simulink model "Controlled_Three_phase_full_wave_bridge_rectifier_PI"  (R2023b)
settings: Solver=VariableStepAuto  StartTime=0.0  StopTime=0.2  RelTol=1e-3
libraries: spsThyristorLib x6, spsSeriesRLCBranchLib x4, spsVoltageMeasurementLib x4, spsACVoltageSourceLib x3, spsCurrentMeasurementLib x1, sps_lib x1
settings Model: Creator=louis  LastModifiedBy=louis

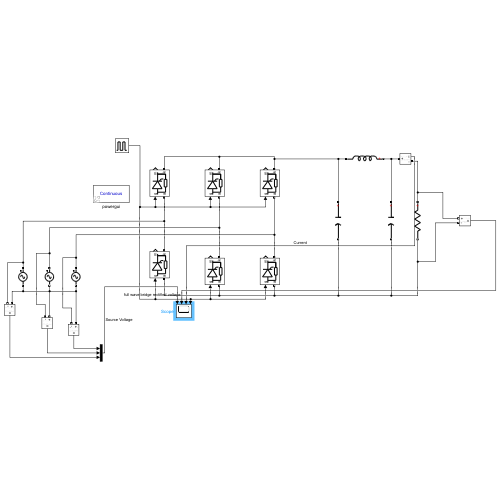
[thumbnail: Simulink's stored preview of the top-level diagram]
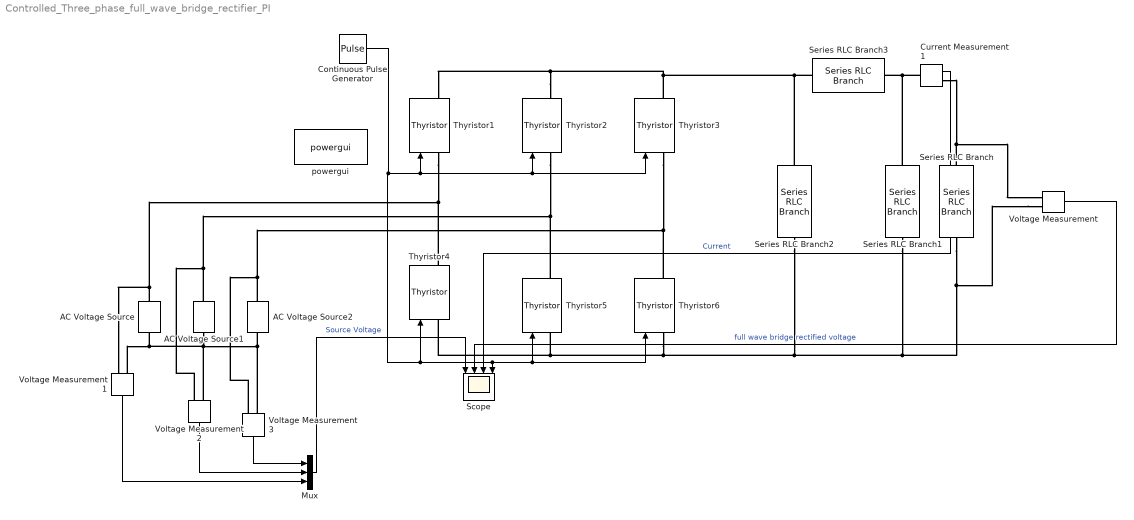
== system Controlled_Three_phase_full_wave_bridge_rectifier_PI ==
  AC Voltage Source : spsACVoltageSourceLib/AC Voltage Source  Amplitude=240  Phase=0  Frequency=50  SampleTime=0  Measurements=None  BusType=swing  Pref=10e3  Qref=0  Qmin=-inf  Qmax=+inf
  AC Voltage Source1 : spsACVoltageSourceLib/AC Voltage Source  Amplitude=240  Phase=120  Frequency=50  SampleTime=0  Measurements=None  BusType=swing  Pref=10e3  Qref=0  Qmin=-inf  Qmax=+inf
  AC Voltage Source2 : spsACVoltageSourceLib/AC Voltage Source  Amplitude=240  Phase=240  Frequency=50  SampleTime=0  Measurements=None  BusType=swing  Pref=10e3  Qref=0  Qmin=-inf  Qmax=+inf
  Continuous Pulse Generator : DiscretePulseGenerator  PulseType=Time based  Period=0.0033  PulseWidth=50  PhaseDelay=0.002
  Current Measurement1 : spsCurrentMeasurementLib/Current Measurement  PhasorSimulation=off  OutputType=Complex  PSBequivalent=0
  Mux : Mux  Inputs=3
  Scope : Scope  NumInputPorts=4
  Series RLC Branch : spsSeriesRLCBranchLib/Series RLC Branch  LConnTagsString=__new0  RConnTagsString=__new0  BranchType=R  Resistance=0.8  Inductance=0.001  SetiL0=off  InitialCurrent=0  Capacitance=1e-6  Setx0=off  InitialVoltage=0  Measurements=None
  Series RLC Branch1 : spsSeriesRLCBranchLib/Series RLC Branch  LConnTagsString=__new0  RConnTagsString=__new0  BranchType=C  Resistance=0.8  Inductance=0.001  SetiL0=off  InitialCurrent=0  Capacitance=0.000001  Setx0=off  InitialVoltage=0  Measurements=None
  Series RLC Branch2 : spsSeriesRLCBranchLib/Series RLC Branch  LConnTagsString=__new0  RConnTagsString=__new0  BranchType=C  Resistance=0.8  Inductance=0.001  SetiL0=off  InitialCurrent=0  Capacitance=0.000001  Setx0=off  InitialVoltage=0  Measurements=None
  Series RLC Branch3 : spsSeriesRLCBranchLib/Series RLC Branch  LConnTagsString=__new0  RConnTagsString=__new0  BranchType=L  Resistance=0.8  Inductance=0.003  SetiL0=off  InitialCurrent=0  Capacitance=0.1  Setx0=off  InitialVoltage=0  Measurements=None
  Thyristor{1..6} (6 alike) : spsThyristorLib/Thyristor  Ron=0.001  Lon=0  Vf=0.8  IC=0  Rs=500  Cs=250e-9  Measurements=on
  Voltage Measurement{,1..3} (4 alike) : spsVoltageMeasurementLib/Voltage Measurement  PhasorSimulation=off  OutputType=Complex  PSBequivalent=0
  powergui : sps_lib/powergui  Priority=1  SimulationMode=Continuous  SampleTime=50e-6  frequency=60  Iterations=50  frequencyindice=0  Pbase=100e6  ErrMax=1e-4  UnitsV=kV  UnitsW=MW  buscounter=0  FunctionMessages=off  echomessages=off  EnableUseOfTLC=off  CurrentSourceSwitches=off  DisableSnubberDevices=off  DisableRonSwitches=off  DisableVfSwitches=off  DisplayEquations=off  AutomaticDiscreteSolvers=off  SolverType=Tustin/Backward Euler (TBE)  Interpol=off  ExternalGateDelay=off  methode=off  Ts=100  x0status=blocks  SPID=on  SwTol=0  HookPort=off  NonlinearTolerance=1e-4  nMaxIteration=100  ContinueOnMaxIteration=off  RestoreLinks=warning  ResistiveCurrentMeasurement=off  Frange=[0:2:500]  Ylog=off  Xlog=on  ShowGrid=off  save=off  variable=ZData  structure=0  ZoomFFT=off  StartTime=0.0  cycles=1  DisplayStyle=1  fundamental=60  FreqAxis=off  MaxFrequency=1000  frequencyindicesteady=1  RmsSteady=1  display=off
  wires:
  Voltage Measurement/1 -> Scope/2  "full wave bridge rectified voltage"
  Voltage Measurement3/1 -> Mux/1
  Voltage Measurement2/1 -> Mux/2
  Voltage Measurement1/1 -> Mux/3
  Mux/1 -> Scope/1  "Source Voltage"
  Continuous Pulse Generator/1 -> Thyristor3/1, Thyristor2/1, Thyristor1/1, Thyristor4/1, Thyristor6/1, Thyristor5/1, Scope/4
  Current Measurement1/1 -> Scope/3  "Current"
  connections:
  Series RLC Branch1/LConn1 -- Series RLC Branch3/LConn1 -- Current Measurement1/LConn1
  Voltage Measurement1/LConn2 -- AC Voltage Source/RConn1 -- Thyristor4/RConn1 -- Thyristor1/LConn1
  Voltage Measurement2/LConn2 -- AC Voltage Source1/RConn1 -- Thyristor5/RConn1 -- Thyristor2/LConn1
  Voltage Measurement/LConn2 -- Series RLC Branch1/RConn1 -- Series RLC Branch2/RConn1 -- Thyristor6/LConn1 -- Thyristor4/LConn1 -- Thyristor5/LConn1 -- Series RLC Branch/RConn1
  Thyristor2/RConn1 -- Series RLC Branch2/LConn1 -- Series RLC Branch3/RConn1 -- Thyristor3/RConn1 -- Thyristor1/RConn1
  Voltage Measurement3/LConn2 -- AC Voltage Source2/RConn1 -- Thyristor6/RConn1 -- Thyristor3/LConn1
  AC Voltage Source1/LConn1 -- Voltage Measurement3/LConn1 -- AC Voltage Source2/LConn1 -- Voltage Measurement2/LConn1 -- Voltage Measurement1/LConn1 -- AC Voltage Source/LConn1
  Series RLC Branch/LConn1 -- Current Measurement1/RConn1 -- Voltage Measurement/LConn1
